simulink model "mc_buffered_mode"  (Simulink 3.0)
libraries: mathlib x15, mc_singlelib x5, genlib x2, analoglib x1, arclib x1

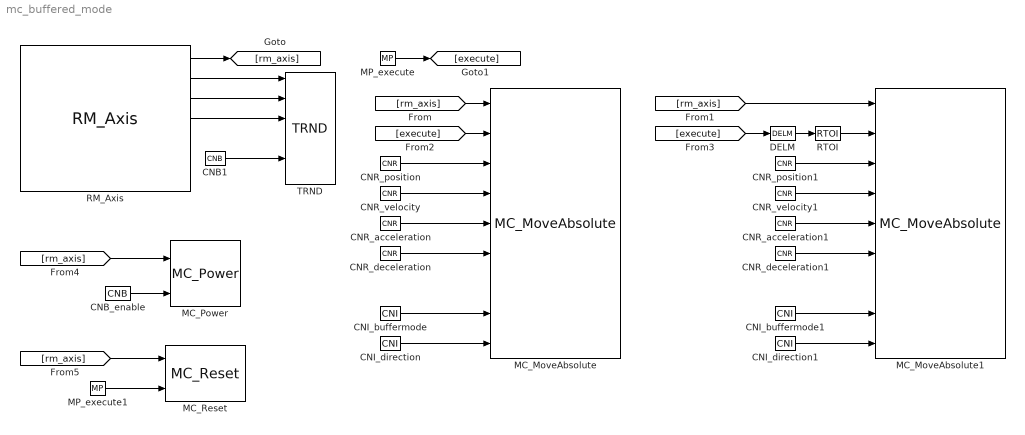
== system mc_buffered_mode ==
  CNB1 : mathlib/CNB  YCN=on
  CNB_enable : mathlib/CNB  SystemSampleTime=-1  YCN=on
  CNI_buffermode : mathlib/CNI  icn=1
  CNI_buffermode1 : mathlib/CNI  icn=1
  CNI_direction : mathlib/CNI  icn=1
  CNI_direction1 : mathlib/CNI  icn=1
  CNR_acceleration : mathlib/CNR  ycn=0.5
  CNR_acceleration1 : mathlib/CNR  ycn=0.5
  CNR_deceleration : mathlib/CNR  ycn=0.5
  CNR_deceleration1 : mathlib/CNR  ycn=0.5
  CNR_position : mathlib/CNR  ycn=10
  CNR_position1 : mathlib/CNR  ycn=20
  CNR_velocity : mathlib/CNR  ycn=1
  CNR_velocity1 : mathlib/CNR  ycn=2
  DELM : analoglib/DELM  del=10  nmax=10000
  MC_MoveAbsolute : mc_singlelib/MC_MoveAbsolute
  MC_MoveAbsolute1 : mc_singlelib/MC_MoveAbsolute
  MC_Power : mc_singlelib/MC_Power  SystemSampleTime=-1
  MC_Reset : mc_singlelib/MC_Reset
  MP_execute : genlib/MP  BSTATE=off  pwidth=1  RPTF=off
  MP_execute1 : genlib/MP  BSTATE=off  pwidth=1  RPTF=off
  RM_Axis : mc_singlelib/RM_Axis  SystemSampleTime=-1  AxisType=1: Linear axis  EnableLimitPos=on  SWLimitPos=1000  MaxPosSystem=1100  EnableLimitNeg=on  SWLimitNeg=-1  MinPosSystem=-2  EnablePosLagMonitor=off  MaxPositionLag=1000  MaxVelocitySystem=600  MaxVelocityAppl=500  MaxAccelerationSystem=1100  MaxAccelerationAppl=1000  MaxDecelerationSystem=1100  MaxDecelerationAppl=1000  MaxJerk=0  MaxTorque=0  kta=0  ReverseLimit=off
  RTOI : mathlib/RTOI
  TRND : arclib/TRND  n=3  l=500  btype=8: Double  ptype1=1: Store  ptype2=1: Store  ptype3=1: Store  ptype4=1: Store  pfac=1  afac=0  arc=0  id=1  Title=Trend Title  timesrc=1
  wires:
  CNB1/1 -> TRND/5
  CNB_enable/1 -> MC_Power/2
  CNI_buffermode/1 -> MC_MoveAbsolute/8
  CNI_buffermode1/1 -> MC_MoveAbsolute1/8
  CNI_direction/1 -> MC_MoveAbsolute/9
  CNI_direction1/1 -> MC_MoveAbsolute1/9
  CNR_acceleration/1 -> MC_MoveAbsolute/5
  CNR_acceleration1/1 -> MC_MoveAbsolute1/5
  CNR_deceleration/1 -> MC_MoveAbsolute/6
  CNR_deceleration1/1 -> MC_MoveAbsolute1/6
  CNR_position/1 -> MC_MoveAbsolute/3
  CNR_position1/1 -> MC_MoveAbsolute1/3
  CNR_velocity/1 -> MC_MoveAbsolute/4
  CNR_velocity1/1 -> MC_MoveAbsolute1/4
  DELM/1 -> RTOI/1
  [rm_axis] -> MC_MoveAbsolute/1
  [rm_axis] -> MC_MoveAbsolute1/1
  [execute] -> MC_MoveAbsolute/2
  [execute] -> DELM/1
  [rm_axis] -> MC_Power/1
  [rm_axis] -> MC_Reset/1
  MP_execute/1 -> [execute]
  MP_execute1/1 -> MC_Reset/2
  RM_Axis/1 -> [rm_axis]
  RM_Axis/2 -> TRND/1
  RM_Axis/3 -> TRND/2
  RM_Axis/4 -> TRND/3
  RTOI/1 -> MC_MoveAbsolute1/2
